simulink model "lab2_DirectDigitalSS_Robust_IntegralAction"  (R2020b)
settings: Solver=VariableStepAuto  StartTime=0.0  StopTime=10.0  RelTol=1e-3
undefined symbols (not defined in the file): DiscIntNeverNeededParam, Gamma0, H0, J0, Ke, Nu, Nx, Phi0, sens, stepAmplitude, Ts
settings Model: Creator=Musta  LastModifiedBy=Musta

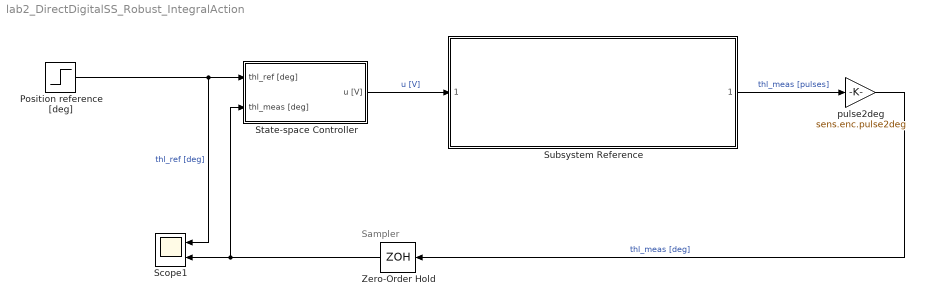
== system lab2_DirectDigitalSS_Robust_IntegralAction ==
  note: Sampler
  Position reference [deg] : Step  Time=0  After=stepAmplitude  SampleTime=0
  Scope1 : Scope  NumInputPorts=2
  State-space Controller : Subsystem
  Subsystem Reference : Subsystem  ReferencedSubsystem=plant_model
  Zero-Order Hold : ZeroOrderHold  SampleTime=Ts
  pulse2deg : Gain  Gain=sens.enc.pulse2deg
  wires:
  Position reference [deg]/1 -> Scope1/1, State-space Controller/1(thl_ref [deg])  "thl_ref [deg]"
  pulse2deg/1 -> Zero-Order Hold/1  "thl_meas [deg]"
  Zero-Order Hold/1 -> Scope1/2, State-space Controller/2(thl_meas [deg])
  State-space Controller/1(u [V]) -> Subsystem Reference/1  "u [V]"
  Subsystem Reference/1 -> pulse2deg/1  "thl_meas [pulses]"

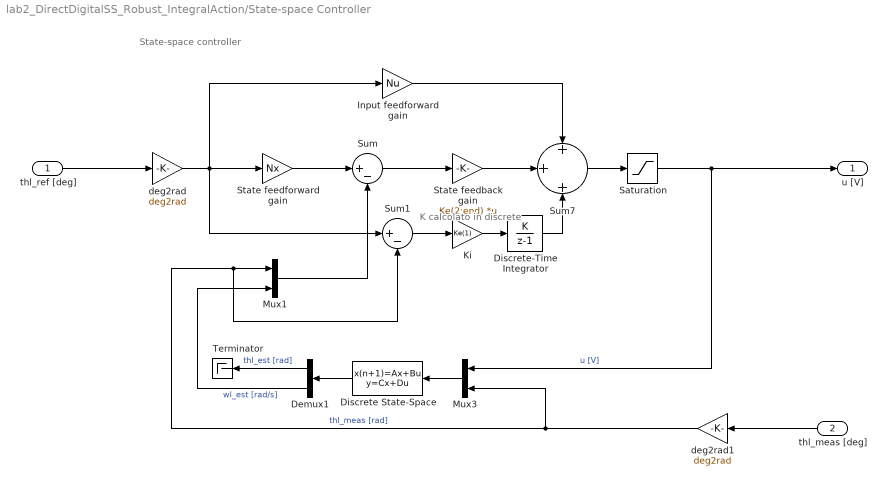
== system lab2_DirectDigitalSS_Robust_IntegralAction/State-space Controller ==
  note: State-space controller
  note: K calcolato in discrete
  thl_ref [deg] : Inport
  thl_meas [deg] : Inport  Port=2
  Demux1 : Demux  Outputs=2
  Discrete State-Space : DiscreteStateSpace  A=Phi0  B=Gamma0  C=H0  D=J0  SampleTime=Ts
  Discrete-Time Integrator : DiscreteIntegrator  IntegratorMethod=Accumulation: Forward Euler  SampleTime=Ts  ICPrevOutput=DiscIntNeverNeededParam  ICPrevScaledInput=DiscIntNeverNeededParam
  Input feedforward gain : Gain  Gain=Nu
  Ki : Gain  Gain=Ke(1)
  Mux1 : Mux  Inputs=2
  Mux3 : Mux  Inputs=2
  Saturation : Saturate  UpperLimit=12  LowerLimit=-12
  "State feedback gain " : Gain  Gain=Ke(2:end)  Multiplication=Matrix(K*u)
  State feedforward gain : Gain  Gain=Nx
  Sum : Sum  Inputs=|+-
  Sum1 : Sum  Inputs=|+-
  Sum7 : Sum  Inputs=+||+||+
  Terminator : Terminator
  deg2rad : Gain  Gain=deg2rad
  deg2rad1 : Gain  Gain=deg2rad
  u [V] : Outport
  wires:
  thl_ref [deg]/1 -> deg2rad/1
  deg2rad/1 -> Sum1/1, Input feedforward gain/1, State feedforward gain/1
  Sum/1 -> "State feedback gain "/1
  State feedforward gain/1 -> Sum/1
  Input feedforward gain/1 -> Sum7/1
  Sum7/1 -> Saturation/1
  Mux1/1 -> Sum/2
  Discrete-Time Integrator/1 -> Sum7/3
  "State feedback gain "/1 -> Sum7/2
  Sum1/1 -> Ki/1
  Ki/1 -> Discrete-Time Integrator/1
  Saturation/1 -> Mux3/1, u [V]/1  "u [V]"
  deg2rad1/1 -> Mux3/2, Sum1/2, Mux1/1  "thl_meas [rad]"
  Demux1/1 -> Terminator/1  "thl_est [rad]"
  Mux3/1 -> Discrete State-Space/1
  Discrete State-Space/1 -> Demux1/1
  thl_meas [deg]/1 -> deg2rad1/1
  Demux1/2 -> Mux1/2  "wl_est [rad/s]"
